simulink model "Test_Piero_23b"  (R2024a)
settings: Solver=VariableStepAuto  StartTime=0.0  StopTime=inf  RelTol=1e-3
settings Model: Creator=m4ttn  LastModifiedBy=m4ttn

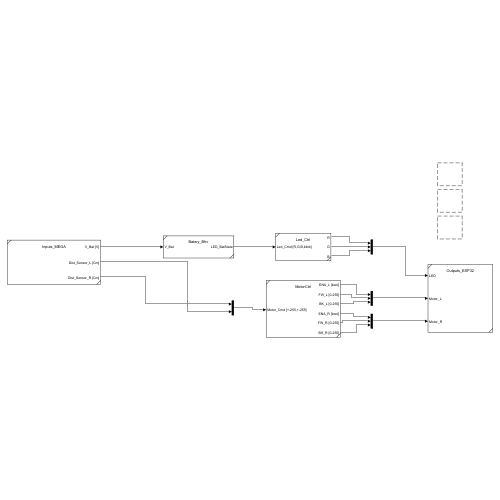
[thumbnail: Simulink's stored preview of the top-level diagram]
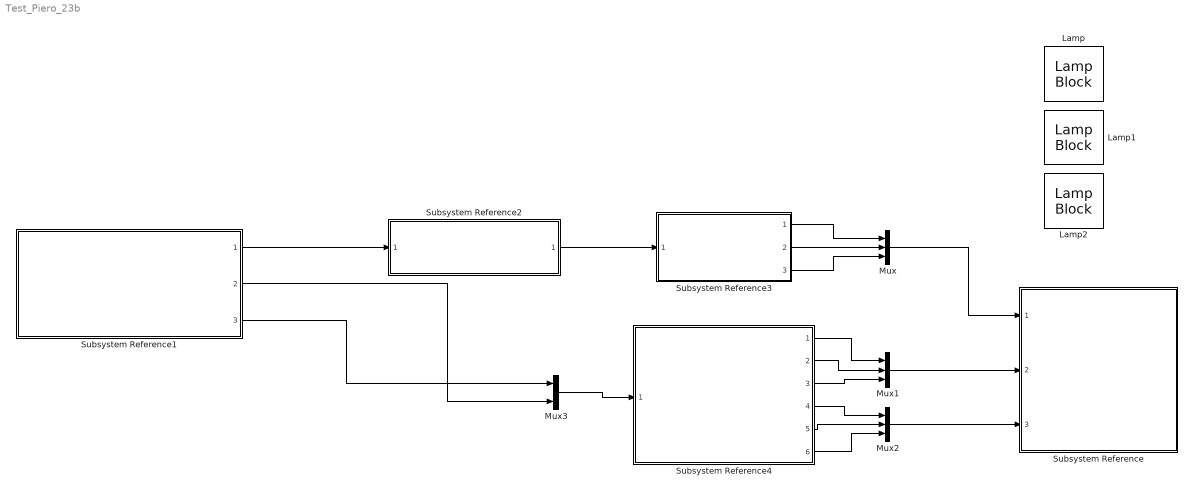
== system Test_Piero_23b ==
  Lamp : LampBlock  LabelPosition=Hide
  Lamp1 : LampBlock  LabelPosition=Hide
  Lamp2 : LampBlock  LabelPosition=Hide
  Mux : Mux  Inputs=3
  Mux1 : Mux  Inputs=3
  Mux2 : Mux  Inputs=3
  Mux3 : Mux  Inputs=2
  Subsystem Reference : Subsystem  ReferencedSubsystem=Outputs_ESP32
  Subsystem Reference1 : Subsystem  ReferencedSubsystem=Inputs_MEGA
  Subsystem Reference2 : Subsystem  ReferencedSubsystem=Batery_Bhv
  Subsystem Reference3 : Subsystem  ReferencedSubsystem=Led_Ctrl
  Subsystem Reference4 : Subsystem  ReferencedSubsystem=MotorCtrl
  wires:
  Subsystem Reference3/1 -> Mux/1
  Subsystem Reference3/2 -> Mux/2
  Subsystem Reference3/3 -> Mux/3
  Mux/1 -> Subsystem Reference/1
  Subsystem Reference4/1 -> Mux1/1
  Subsystem Reference4/2 -> Mux1/2
  Subsystem Reference4/3 -> Mux1/3
  Subsystem Reference4/4 -> Mux2/1
  Subsystem Reference4/5 -> Mux2/2
  Subsystem Reference4/6 -> Mux2/3
  Mux1/1 -> Subsystem Reference/2
  Mux2/1 -> Subsystem Reference/3
  Subsystem Reference2/1 -> Subsystem Reference3/1
  Mux3/1 -> Subsystem Reference4/1
  Subsystem Reference1/1 -> Subsystem Reference2/1
  Subsystem Reference1/3 -> Mux3/1
  Subsystem Reference1/2 -> Mux3/2
